simulink model "adative_HW_4_1"  (R2015a)
settings: Solver=ode45  StartTime=0.0  StopTime=50  MaxStep=0.1  MinStep=0.0001  RelTol=1e-3  AbsTol=1e-3
settings Model: Creator=Hybrid Pederson  LastModifiedBy=ccpc50
settings DataIOCC: SignalLoggingSaveFormat=ModelDataLogs  SaveOutput=off  SaveTime=off
settings OptimizationCC: ExpressionDepthLimit=2147483647  InitFltsAndDblsToZero=on
settings DebuggingCC: SaveWithParameterizedLinksMsg=none  UnderspecifiedInitializationDetection=Classic  MergeDetectMultiDrivingBlocksExec=none  SolverPrmCheckMsg=warning  FcnCallInpInsideContextMsg=UseLocalSettings  StateNameClashWarn=warning
settings GRTTargetCC: TargetFcnLib=ansi_tfl_tmw.mat  CombineOutputUpdateFcns=off  GRTInterface=on

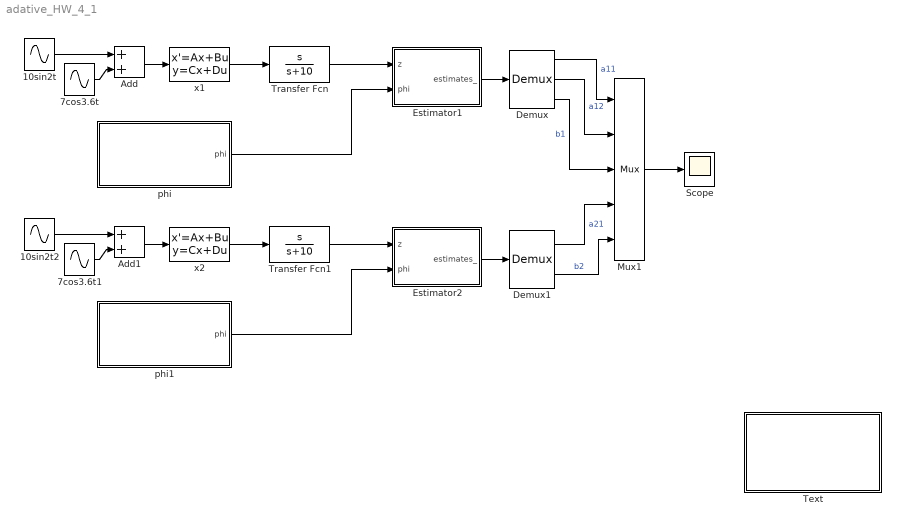
== system adative_HW_4_1 ==
  10sin2t : Sin  Amplitude=10  Frequency=2
  10sin2t2 : Sin  Amplitude=10  Frequency=2
  7cos3.6t : Sin  Amplitude=7  Frequency=3.6  Phase=90
  7cos3.6t1 : Sin  Amplitude=7  Frequency=3.6  Phase=90
  Add : Sum
  Add1 : Sum
  Demux : Demux  Outputs=3
  Demux1 : Demux  Outputs=2
  Estimator1 : Subsystem
      mask Display: disp('Parameter\nEstimation')
  Estimator2 : Subsystem
      mask Display: disp('Parameter\nEstimation')
  Mux1 : Mux  Inputs=5
  Scope : Scope
      settings: TickLabels=on  ShowLegends=on
  Text : Subsystem
      mask Display: disp('Double click here\nfor help to run\nthe simulation')
  Transfer Fcn : TransferFcn  Numerator=[1 0]  Denominator=[1 10]
  Transfer Fcn1 : TransferFcn  Numerator=[1 0]  Denominator=[1 10]
  phi : Subsystem
      mask Display: disp('phi=[sinwt coswt]')
  phi1 : Subsystem
      mask Display: disp('phi=[sinwt coswt]')
  x1 : StateSpace  A=[-0.25 3; -5 0]  B=[1; 2.2]  C=[1 0]  D=0  X0=0
  x2 : StateSpace  A=[-0.25 3; -5 0]  B=[1; 2.2]  C=[0 1]  D=0  X0=0
  wires:
  phi/1(phi) -> Estimator1/2(phi)
  x1/1 -> Transfer Fcn/1
  Transfer Fcn/1 -> Estimator1/1(z)
  phi1/1(phi) -> Estimator2/2(phi)
  x2/1 -> Transfer Fcn1/1
  Transfer Fcn1/1 -> Estimator2/1(z)
  Estimator1/1(estimates_) -> Demux/1
  Estimator2/1(estimates_) -> Demux1/1
  Demux/1 -> Mux1/1  "a11"
  Demux/3 -> Mux1/3  "b1"
  Demux/2 -> Mux1/2  "a12"
  Demux1/1 -> Mux1/4  "a21"
  Demux1/2 -> Mux1/5  "b2"
  Mux1/1 -> Scope/1
  10sin2t/1 -> Add/1
  7cos3.6t/1 -> Add/2
  Add/1 -> x1/1
  10sin2t2/1 -> Add1/1
  7cos3.6t1/1 -> Add1/2
  Add1/1 -> x2/1

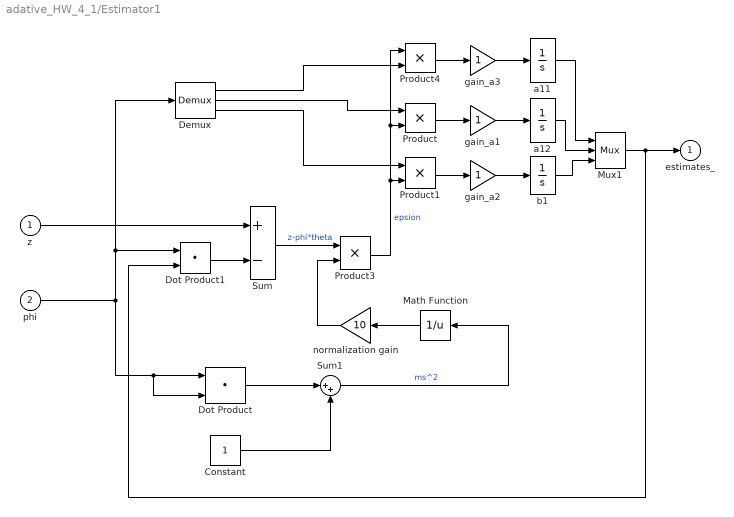
== system adative_HW_4_1/Estimator1 ==
  z : Inport
  phi : Inport  Port=2
  Constant : Constant
  Demux : Demux  Outputs=3
  Dot Product : DotProduct  InputSameDT=on  OutDataTypeStr=Inherit: Inherit via internal rule
  Dot Product1 : DotProduct  InputSameDT=on  OutDataTypeStr=Inherit: Inherit via internal rule
  Math Function : Math  Operator=reciprocal  SaturateOnIntegerOverflow=on
  Mux1 : Mux  Inputs=3
  Product{,1,3..4} (4 alike) : Product  SaturateOnIntegerOverflow=on  RndMeth=Zero  InputSameDT=on  OutDataTypeStr=Inherit: Same as first input
  Sum : Sum  Inputs=+-  SaturateOnIntegerOverflow=on  InputSameDT=on  OutDataTypeStr=Inherit: Same as first input
  Sum1 : Sum  Inputs=|++
  a11 : Integrator
  a12 : Integrator
  b1 : Integrator
  gain_a1 : Gain  SaturateOnIntegerOverflow=on  OutDataTypeStr=Inherit: Same as input  ParamDataTypeStr=Inherit: Same as input
  gain_a2 : Gain  SaturateOnIntegerOverflow=on  OutDataTypeStr=Inherit: Same as input  ParamDataTypeStr=Inherit: Same as input
  gain_a3 : Gain  SaturateOnIntegerOverflow=on  OutDataTypeStr=Inherit: Same as input  ParamDataTypeStr=Inherit: Same as input
  normalization gain : Gain  Gain=10  SaturateOnIntegerOverflow=on  OutDataTypeStr=Inherit: Same as input  ParamDataTypeStr=Inherit: Same as input
  estimates_ : Outport
  wires:
  z/1 -> Sum/1
  normalization gain/1 -> Product3/2
  Mux1/1 -> Dot Product1/2, estimates_/1
  Math Function/1 -> normalization gain/1
  Product1/1 -> gain_a2/1
  gain_a2/1 -> b1/1
  Product/1 -> gain_a1/1
  gain_a1/1 -> a12/1
  Dot Product1/1 -> Sum/2
  Product3/1 -> Product4/1, Product/2, Product1/2  "epsion"
  Sum/1 -> Product3/1  "z-phi*theta"
  phi/1 -> Demux/1, Dot Product1/1, Dot Product/2, Dot Product/1
  gain_a3/1 -> a11/1
  Product4/1 -> gain_a3/1
  Demux/1 -> Product4/2
  Demux/2 -> Product/1
  Demux/3 -> Product1/1
  Dot Product/1 -> Sum1/1
  Constant/1 -> Sum1/2
  Sum1/1 -> Math Function/1  "ms^2"
  a11/1 -> Mux1/1
  a12/1 -> Mux1/2
  b1/1 -> Mux1/3

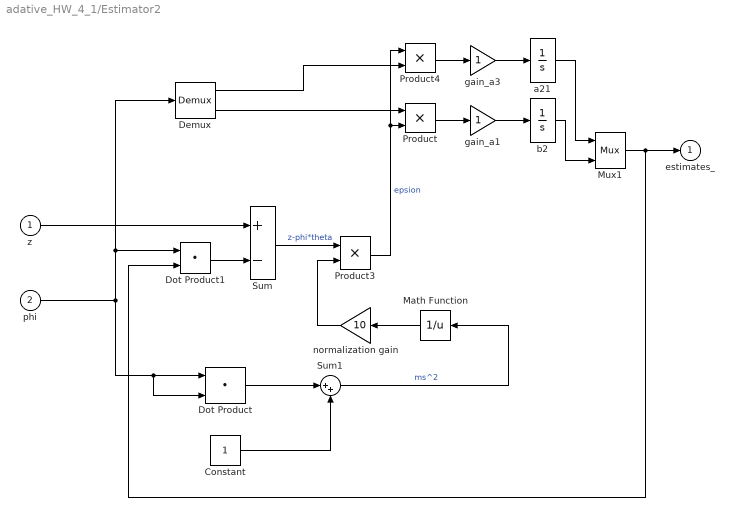
== system adative_HW_4_1/Estimator2 ==
  z : Inport
  phi : Inport  Port=2
  Constant : Constant
  Demux : Demux  Outputs=2
  Dot Product : DotProduct  InputSameDT=on  OutDataTypeStr=Inherit: Inherit via internal rule
  Dot Product1 : DotProduct  InputSameDT=on  OutDataTypeStr=Inherit: Inherit via internal rule
  Math Function : Math  Operator=reciprocal  SaturateOnIntegerOverflow=on
  Mux1 : Mux  Inputs=2
  Product : Product  SaturateOnIntegerOverflow=on  RndMeth=Zero  InputSameDT=on  OutDataTypeStr=Inherit: Same as first input
  Product3 : Product  SaturateOnIntegerOverflow=on  RndMeth=Zero  InputSameDT=on  OutDataTypeStr=Inherit: Same as first input
  Product4 : Product  SaturateOnIntegerOverflow=on  RndMeth=Zero  InputSameDT=on  OutDataTypeStr=Inherit: Same as first input
  Sum : Sum  Inputs=+-  SaturateOnIntegerOverflow=on  InputSameDT=on  OutDataTypeStr=Inherit: Same as first input
  Sum1 : Sum  Inputs=|++
  a21 : Integrator
  b2 : Integrator
  gain_a1 : Gain  SaturateOnIntegerOverflow=on  OutDataTypeStr=Inherit: Same as input  ParamDataTypeStr=Inherit: Same as input
  gain_a3 : Gain  SaturateOnIntegerOverflow=on  OutDataTypeStr=Inherit: Same as input  ParamDataTypeStr=Inherit: Same as input
  normalization gain : Gain  Gain=10  SaturateOnIntegerOverflow=on  OutDataTypeStr=Inherit: Same as input  ParamDataTypeStr=Inherit: Same as input
  estimates_ : Outport
  wires:
  z/1 -> Sum/1
  normalization gain/1 -> Product3/2
  Mux1/1 -> Dot Product1/2, estimates_/1
  Math Function/1 -> normalization gain/1
  Product/1 -> gain_a1/1
  gain_a1/1 -> b2/1
  Dot Product1/1 -> Sum/2
  Product3/1 -> Product4/1, Product/2  "epsion"
  Sum/1 -> Product3/1  "z-phi*theta"
  phi/1 -> Demux/1, Dot Product1/1, Dot Product/2, Dot Product/1
  gain_a3/1 -> a21/1
  Product4/1 -> gain_a3/1
  Demux/1 -> Product4/2
  Demux/2 -> Product/1
  Dot Product/1 -> Sum1/1
  Constant/1 -> Sum1/2
  Sum1/1 -> Math Function/1  "ms^2"
  a21/1 -> Mux1/1
  b2/1 -> Mux1/2

== system adative_HW_4_1/Text ==
  note: 4) The noise level (the gain in the Noise Source block)
  note: 3) The transfer function W(s) in the receiver and in the
      | Estimator block
  note: 2) The normalization gain alpha in the Estimator block
  note: 1) The adaptive gain (gain_a1, gain_a2 in the Estimator block)
  note: You can use Start/Stop in the Simulation pull-down
      | menu to run the program. Or you can change the
      | following parameters to see how they affect the
      | simulation results:

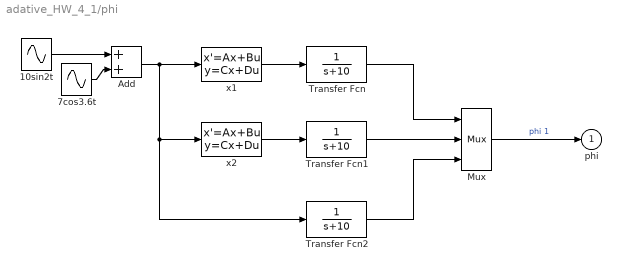
== system adative_HW_4_1/phi ==
  10sin2t : Sin  Amplitude=10  Frequency=2
  7cos3.6t : Sin  Amplitude=7  Frequency=3.6  Phase=90
  Add : Sum
  Mux : Mux  Inputs=3
  Transfer Fcn : TransferFcn  Denominator=[1 10]
  Transfer Fcn1 : TransferFcn  Denominator=[1 10]
  Transfer Fcn2 : TransferFcn  Denominator=[1 10]
  x1 : StateSpace  A=[-0.25 3; -5 0]  B=[1; 2.2]  C=[1 0]  D=0  X0=0
  x2 : StateSpace  A=[-0.25 3; -5 0]  B=[1; 2.2]  C=[0 1]  D=0  X0=0
  phi : Outport
  wires:
  Mux/1 -> phi/1  "phi 1"
  Add/1 -> Transfer Fcn2/1, x2/1, x1/1
  x1/1 -> Transfer Fcn/1
  x2/1 -> Transfer Fcn1/1
  Transfer Fcn/1 -> Mux/1
  Transfer Fcn1/1 -> Mux/2
  Transfer Fcn2/1 -> Mux/3
  10sin2t/1 -> Add/1
  7cos3.6t/1 -> Add/2

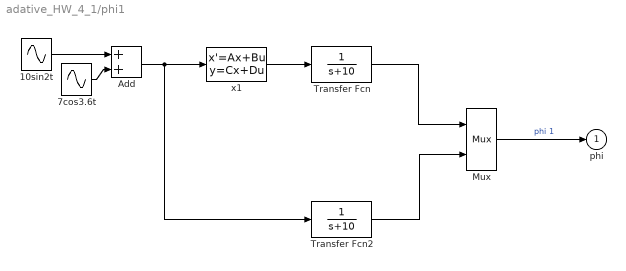
== system adative_HW_4_1/phi1 ==
  10sin2t : Sin  Amplitude=10  Frequency=2
  7cos3.6t : Sin  Amplitude=7  Frequency=3.6  Phase=90
  Add : Sum
  Mux : Mux  Inputs=2
  Transfer Fcn : TransferFcn  Denominator=[1 10]
  Transfer Fcn2 : TransferFcn  Denominator=[1 10]
  x1 : StateSpace  A=[-0.25 3; -5 0]  B=[1; 2.2]  C=[1 0]  D=0  X0=0
  phi : Outport
  wires:
  Mux/1 -> phi/1  "phi 1"
  Add/1 -> Transfer Fcn2/1, x1/1
  x1/1 -> Transfer Fcn/1
  Transfer Fcn/1 -> Mux/1
  Transfer Fcn2/1 -> Mux/2
  10sin2t/1 -> Add/1
  7cos3.6t/1 -> Add/2
